simulink model "W05_1_vrx"  (R2024b)
settings: Solver=ode4  StartTime=0.0  StopTime=inf  FixedStep=Ts_ctrl  RelTol=1e-3
values from neighbouring files (symbols this model uses):
  animate = 0    [W05_compare.m]    (also in W05_crab_demo.m; W05_lookahead_demo.m; W05_setup.m = 1; W07_setup.m = 1)
  Delta = DELTAS(i)    [W05_lookahead_demo.m]    (also in W05_setup.m = 10; W07_setup.m = 10)
  F_max = 500    [W05_setup.m]    (also in W07_setup.m)
  guidance_mode = CASES{i,2}    [W05_compare.m]    (also in W05_setup.m = 2; W07_setup.m = 2)
  half_beam = 1.027135    [W05_setup.m]    (also in W07_setup.m)
  k_prop = 1000 * 0.004422 * 0.2^4    (= 0.0070752)    [W05_setup.m]    (also in W07_setup.m)
  Kd_psi = 200    [W05_setup.m]    (also in W07_setup.m)
  Ki_u = 100    [W05_setup.m]    (also in W07_setup.m)
  Kp_psi = 400    [W05_setup.m]    (also in W07_setup.m)
  Kp_u = 300    [W05_setup.m]    (also in W07_setup.m)
  n_max = sqrt(F_max / k_prop)    [W05_setup.m]    (also in W07_setup.m)
  origin_east = -532    [W05_setup.m]    (also in W07_setup.m)
  origin_north = 162    [W05_setup.m]    (also in W07_setup.m)
  R_LOS = 5    [W05_lookahead_demo.m]    (also in W05_setup.m; W07_setup.m)
  sw_mode = 1    [W05_lookahead_demo.m]    (also in W05_setup.m; W07_setup.m)
  tau_n = 0.30    (= 0.3)    [W05_setup.m]    (also in W07_setup.m)
  Ts_ctrl = 0.05    [W05_setup.m]    (also in W07_setup.m)
  u_ref = 1.5    [W05_setup.m]    (also in W07_setup.m)
  wp_east = [  20   20  100  100   20 ]    [W05_setup.m]    (also in W07_setup.m)
  wp_north = [ -20   60   60  -20  -20 ]    [W05_setup.m]    (also in W07_setup.m)
libraries: ros2lib x5, slpidlib x1
settings Model: Creator=admin  LastModifiedBy=admin

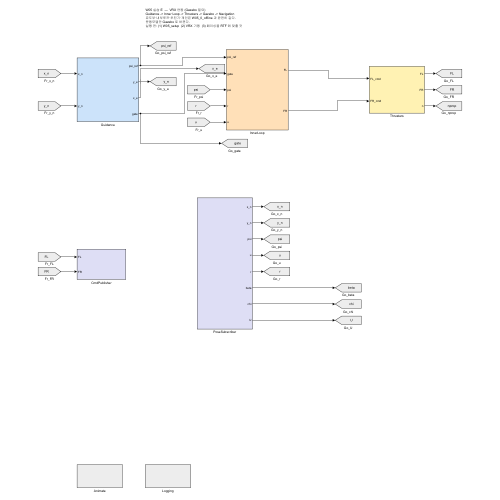
[thumbnail: Simulink's stored preview of the top-level diagram]
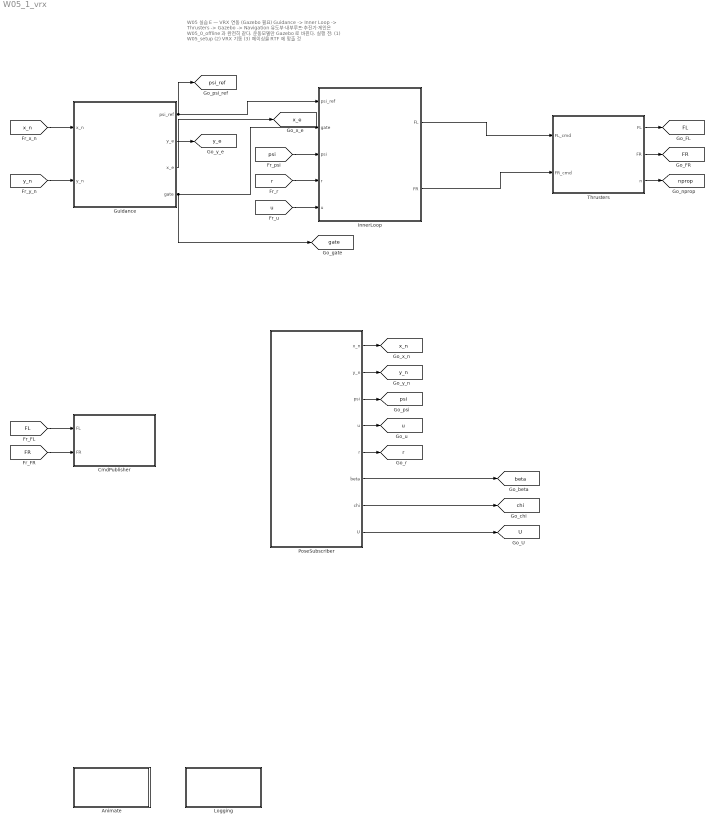
== system W05_1_vrx ==
  note: W05 실습 E  —  VRX 연동 (Gazebo 필요)
      | Guidance -> Inner Loop -> Thrusters -> Gazebo -> Navigation
      | 유도부·내부루프·추진기·게인은 W05_0_offline 과 완전히 같다.
      | 운동모델만 Gazebo 로 바뀐다.
      | 실행 전: (1) W05_setup  (2) VRX 기동  (3) 페이싱을 RTF 에 맞출 것
  Animate : Subsystem
  CmdPublisher : Subsystem
  Guidance : Subsystem
  InnerLoop : Subsystem
  Logging : Subsystem
  PoseSubscriber : Subsystem
  Thrusters : Subsystem
  tag scope: FL=global, FR=global, U=global, beta=global, chi=global, gate=global, nprop=global, psi=global, psi_ref=global, r=global, u=global, x_e=global, x_n=global, y_e=global, y_n=global
  wires:
  [FR] -> CmdPublisher/2(FR)
  [FL] -> CmdPublisher/1(FL)
  InnerLoop/2(FR) -> Thrusters/2(FR_cmd)
  InnerLoop/1(FL) -> Thrusters/1(FL_cmd)
  [u] -> InnerLoop/5(u)
  [r] -> InnerLoop/4(r)
  [psi] -> InnerLoop/3(psi)
  Guidance/4(gate) -> InnerLoop/2(gate), [gate]
  Guidance/1(psi_ref) -> InnerLoop/1(psi_ref), [psi_ref]
  [y_n] -> Guidance/2(y_n)
  [x_n] -> Guidance/1(x_n)
  Thrusters/1(FL) -> [FL]
  Thrusters/2(FR) -> [FR]
  PoseSubscriber/8(U) -> [U]
  PoseSubscriber/6(beta) -> [beta]
  PoseSubscriber/7(chi) -> [chi]
  Thrusters/3(n) -> [nprop]
  PoseSubscriber/3(psi) -> [psi]
  PoseSubscriber/5(r) -> [r]
  PoseSubscriber/4(u) -> [u]
  Guidance/3(x_e) -> [x_e]
  PoseSubscriber/1(x_n) -> [x_n]
  Guidance/2(y_e) -> [y_e]
  PoseSubscriber/2(y_n) -> [y_n]

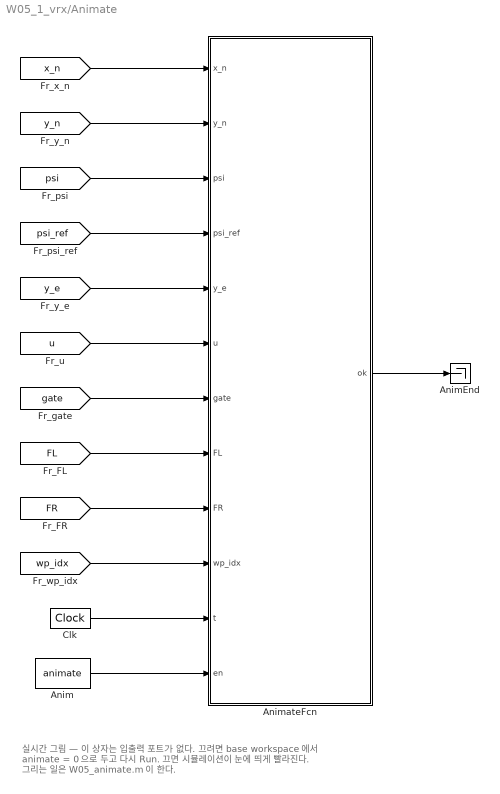
== system W05_1_vrx/Animate ==
  note: 실시간 그림 — 이 상자는 입출력 포트가 없다.
      | 끄려면 base workspace 에서  animate = 0  으로 두고 다시 Run.
      | 끄면 시뮬레이션이 눈에 띄게 빨라진다.
      | 그리는 일은 W05_animate.m 이 한다.
  Anim : Constant  Value=animate
  AnimEnd : Terminator
  AnimateFcn : MATLAB Function  TreatAsAtomicUnit=on
  Clk : DigitalClock  SampleTime=Ts_ctrl
  wires:
  [x_n] -> AnimateFcn/1(x_n)
  [y_n] -> AnimateFcn/2(y_n)
  [psi] -> AnimateFcn/3(psi)
  [psi_ref] -> AnimateFcn/4(psi_ref)
  [y_e] -> AnimateFcn/5(y_e)
  [u] -> AnimateFcn/6(u)
  [gate] -> AnimateFcn/7(gate)
  [FL] -> AnimateFcn/8(FL)
  [FR] -> AnimateFcn/9(FR)
  [wp_idx] -> AnimateFcn/10(wp_idx)
  Clk/1 -> AnimateFcn/11(t)
  Anim/1 -> AnimateFcn/12(en)
  AnimateFcn/1(ok) -> AnimEnd/1

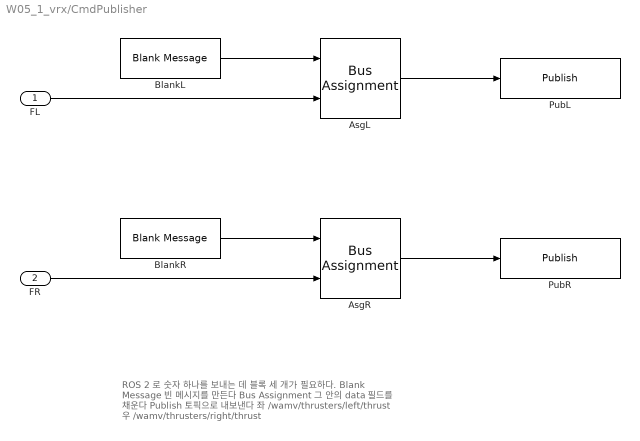
== system W05_1_vrx/CmdPublisher ==
  note: ROS 2 로 숫자 하나를 보내는 데 블록 세 개가 필요하다.
      |   Blank Message   빈 메시지를 만든다
      |   Bus Assignment  그 안의 data 필드를 채운다
      |   Publish         토픽으로 내보낸다
      |
      | 좌 /wamv/thrusters/left/thrust
      | 우 /wamv/thrusters/right/thrust
  FL : Inport
  FR : Inport  Port=2
  AsgL : BusAssignment  AssignedSignals=data
  AsgR : BusAssignment  AssignedSignals=data
  BlankL : ros2lib/Blank Message  messageClass=Message  entityType=std_msgs/Float64  messageType=std_msgs/Float64  SampleTime=Ts_ctrl
  BlankR : ros2lib/Blank Message  messageClass=Message  entityType=std_msgs/Float64  messageType=std_msgs/Float64  SampleTime=Ts_ctrl
  PubL : ros2lib/Publish  topicSource=Specify your own  topic=/wamv/thrusters/left/thrust  messageType=std_msgs/Float64  QOSHistory=Keep last  QOSDepth=1  QOSReliability=Reliable  QOSDurability=Volatile  QOSDeadline=Inf  QOSLifespan=Inf  QOSLiveliness=Automatic  QOSLeaseDuration=Inf  QOSAvoidROSNamespaceConventions=off
  PubR : ros2lib/Publish  topicSource=Specify your own  topic=/wamv/thrusters/right/thrust  messageType=std_msgs/Float64  QOSHistory=Keep last  QOSDepth=1  QOSReliability=Reliable  QOSDurability=Volatile  QOSDeadline=Inf  QOSLifespan=Inf  QOSLiveliness=Automatic  QOSLeaseDuration=Inf  QOSAvoidROSNamespaceConventions=off
  wires:
  BlankL/1 -> AsgL/1
  AsgL/1 -> PubL/1
  FL/1 -> AsgL/2
  BlankR/1 -> AsgR/1
  AsgR/1 -> PubR/1
  FR/1 -> AsgR/2

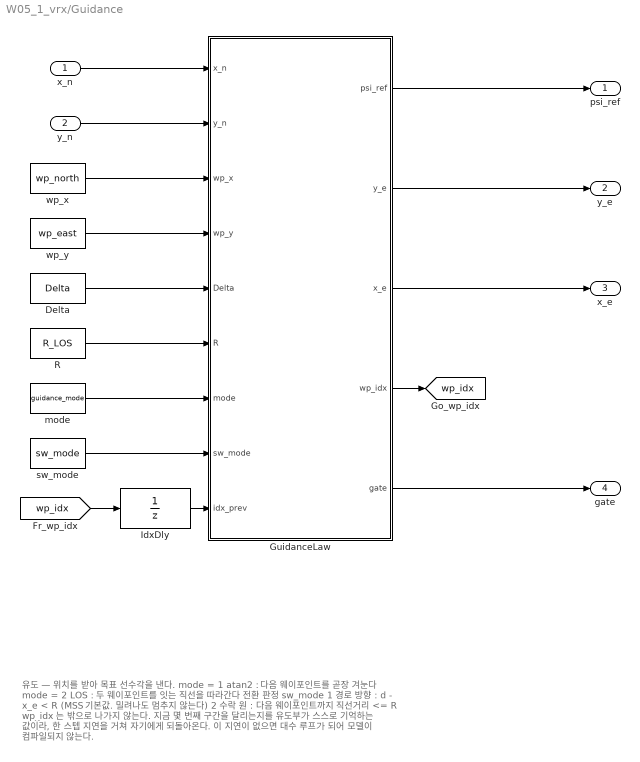
== system W05_1_vrx/Guidance ==
  note: 유도 — 위치를 받아 목표 선수각을 낸다.
      |   mode = 1  atan2 : 다음 웨이포인트를 곧장 겨눈다
      |   mode = 2  LOS   : 두 웨이포인트를 잇는 직선을 따라간다
      |
      | 전환 판정 sw_mode
      |   1  경로 방향 : d - x_e < R   (MSS 기본값. 밀려나도 멈추지 않는다)
      |   2  수락 원   : 다음 웨이포인트까지 직선거리 <= R
      |
      | wp_idx 는 밖으로 나가지 않는다. 지금 몇 번째 구간을 달리는지를
      | 유도부가 스스로 기억하는 값이라, 한 스텝 지연을 거쳐 자기에게 되돌아온다.
      | 이 지연이 없으면 대수 루프가 되어 모델이 컴파일되지 않는다.
  x_n : Inport
  y_n : Inport  Port=2
  Delta : Constant  Value=Delta
  GuidanceLaw : MATLAB Function  TreatAsAtomicUnit=on
  IdxDly : UnitDelay  Description=대수 루프 차단 + 사건 계수기 — 웨이포인트 번호는 정수이고, 유도부가 낸 값이 유도부로 되돌아온다. 미분방정식의 상태가 아니다.  InitialCondition=1  SampleTime=Ts_ctrl  HasFrameUpgradeWarning=on
  R : Constant  Value=R_LOS
  mode : Constant  Value=guidance_mode
  sw_mode : Constant  Value=sw_mode
  wp_x : Constant  Value=wp_north
  wp_y : Constant  Value=wp_east
  psi_ref : Outport
  y_e : Outport  Port=2
  x_e : Outport  Port=3
  gate : Outport  Port=4
  tag scope: wp_idx=global
  wires:
  x_n/1 -> GuidanceLaw/1(x_n)
  y_n/1 -> GuidanceLaw/2(y_n)
  wp_x/1 -> GuidanceLaw/3(wp_x)
  wp_y/1 -> GuidanceLaw/4(wp_y)
  Delta/1 -> GuidanceLaw/5(Delta)
  R/1 -> GuidanceLaw/6(R)
  mode/1 -> GuidanceLaw/7(mode)
  sw_mode/1 -> GuidanceLaw/8(sw_mode)
  [wp_idx] -> IdxDly/1
  IdxDly/1 -> GuidanceLaw/9(idx_prev)
  GuidanceLaw/1(psi_ref) -> psi_ref/1
  GuidanceLaw/2(y_e) -> y_e/1
  GuidanceLaw/3(x_e) -> x_e/1
  GuidanceLaw/5(gate) -> gate/1
  GuidanceLaw/4(wp_idx) -> [wp_idx]

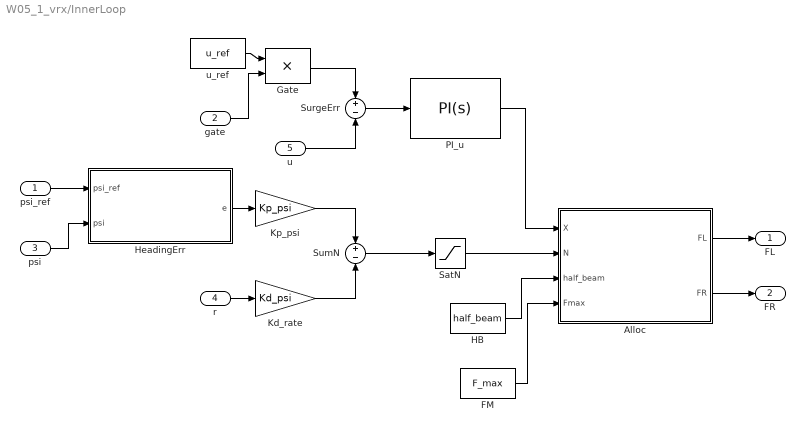
== system W05_1_vrx/InnerLoop ==
  psi_ref : Inport
  gate : Inport  Port=2
  psi : Inport  Port=3
  r : Inport  Port=4
  u : Inport  Port=5
  Alloc : MATLAB Function  TreatAsAtomicUnit=on
  FM : Constant  Value=F_max
  Gate : Product
  HB : Constant  Value=half_beam
  HeadingErr : MATLAB Function  TreatAsAtomicUnit=on
  Kd_rate : Gain  Gain=Kd_psi
  Kp_psi : Gain  Gain=Kp_psi
  PI_u : slpidlib/PID Controller  Controller=PI  Form=Parallel  TimeDomain=Continuous-time  UseExternalTs=off  SampleTime=-1  IntegratorMethod=Forward Euler  FilterMethod=Forward Euler  ControllerParametersSource=internal  P=Kp_u  I=Ki_u  UseKiTs=off  D=0  UseExternalDerivativeSource=off  N=100  UseFilter=on  TunerSelectOption=Transfer Function Based (PID Tuner App)  InitialConditionSource=internal  InitialConditionForIntegrator=0  InitialConditionForFilter=0  DifferentiatorICPrevScaledInput=0  ExternalReset=none  TrackingMode=off  Kt=1  LimitOutput=on  SatLimitsSource=internal  UpperSaturationLimit=2*F_max  LowerSaturationLimit=-2*F_max  LinearizeAsGain=on  AntiWindupMode=clamping  Kb=1  LimitIntegrator=off  UpperIntegratorSaturationLimit=inf  LowerIntegratorSaturationLimit=-inf  POutMin=[]  POutMax=[]  IOutMin=[]  IOutMax=[]  DOutMin=[]  DOutMax=[]  NOutMin=[]  NOutMax=[]  SumOutMin=[]  SumOutMax=[]  SaturationOutMin=[]  SaturationOutMax=[]  PParamMin=[]  PParamMax=[]  IParamMin=[]  IParamMax=[]  DParamMin=[]  DParamMax=[]  NParamMin=[]  NParamMax=[]  KbParamMin=[]  KbParamMax=[]  KtParamMin=[]  KtParamMax=[]  KbOutMin=[]  KbOutMax=[]  KtOutMin=[]  KtOutMax=[]  IntegratorOutMin=[]  IntegratorOutMax=[]  FilterOutMin=[]  FilterOutMax=[]  SumI1OutMin=[]  SumI1OutMax=[]  SumI2OutMin=[]  SumI2OutMax=[]  SumI3OutMin=[]  SumI3OutMax=[]  SumI4OutMin=[]  SumI4OutMax=[]  SumDOutMin=[]  SumDOutMax=[]  DifferentiatorOutMin=[]  DifferentiatorOutMax=[]  FilterDiffOutCoefMin=[]  FilterDiffOutCoefMax=[]  ReciprocalOutMin=[]  ReciprocalOutMax=[]  SumDenOutMin=[]  SumDenOutMax=[]  SumNumOutMin=[]  SumNumOutMax=[]  DivideOutMin=[]  DivideOutMax=[]  UdiffTsProdOutMin=[]  UdiffTsProdOutMax=[]  NTsProdOutMin=[]  NTsProdOutMax=[]  UintegralTsProdOutMin=[]  UintegralTsProdOutMax=[]  UngainTsProdOutMin=[]  UngainTsProdOutMax=[]  ClampingZeroOutDataTypeStr=Inherit: Inherit via back propagation  ClampingZeroOutMin=[]  ClampingZeroOutMax=[]  FilterDenConstantOutDataTypeStr=Inherit: Inherit via back propagation  FilterDenConstantOutMin=[]  FilterDenConstantOutMax=[]  PCopyOutDataTypeStr=Inherit: Inherit via back propagation  PCopyOutMin=[]  PCopyOutMax=[]  NCopyOutDataTypeStr=Inherit: Inherit via back propagation  NCopyOutMin=[]  NCopyOutMax=[]  IntegratorContinuousStateAttributes=''  IntegratorStateMustResolveToSignalObject=off  IntegratorRTWStateStorageClass=Auto  FilterContinuousStateAttributes=''  FilterStateMustResolveToSignalObject=off  FilterRTWStateStorageClass=Auto  ParallelPVariant=InternalParameters  IdealPVariant=Disabled  IVariant=InternalParameters  DVariant=Disabled  IntegratorVariant=Continuous  SatVariant=Enabled  AWVariant=ContClampingParallel  PCopyVariant=Disabled  TRVariant=Disabled  FdbkBlocksVariant=Forward  IdealPFdbkVariant=Disabled  SatFdbkVariant=Disabled  DerivativeFilterVariant=Disabled  NVariant=Disabled  NCopyVariant=Disabled_SignalSpec  FilterICVariant=Disabled  IntegratorICVariant=InternalICs  ExternalResetVariant=Disabled  TRSumVariant=Passthrough  SumFdbkVariant=Disabled  SumVariant=Sum_PI  TsampFilterVariant=InternalTs  TsampNgainVariant=Passthrough  TsampIntegralVariant=Disabled_SignalSpec  ExternalSaturationOutDataTypeStr=Inherit: Same as second input  DerivativeSourceVariant=Disabled  PreIntVariant=InternalPreInt
  SatN : Saturate  UpperLimit=2*F_max*half_beam  LowerLimit=-2*F_max*half_beam
  SumN : Sum  Inputs=+-
  SurgeErr : Sum  Inputs=+-
  u_ref : Constant  Value=u_ref
  FL : Outport
  FR : Outport  Port=2
  wires:
  psi_ref/1 -> HeadingErr/1(psi_ref)
  HeadingErr/1(e) -> Kp_psi/1
  u/1 -> SurgeErr/2
  Gate/1 -> SurgeErr/1
  psi/1 -> HeadingErr/2(psi)
  u_ref/1 -> Gate/1
  HB/1 -> Alloc/3(half_beam)
  gate/1 -> Gate/2
  r/1 -> Kd_rate/1
  Kp_psi/1 -> SumN/1
  Kd_rate/1 -> SumN/2
  SurgeErr/1 -> PI_u/1
  SumN/1 -> SatN/1
  PI_u/1 -> Alloc/1(X)
  SatN/1 -> Alloc/2(N)
  FM/1 -> Alloc/4(Fmax)
  Alloc/1(FL) -> FL/1
  Alloc/2(FR) -> FR/1

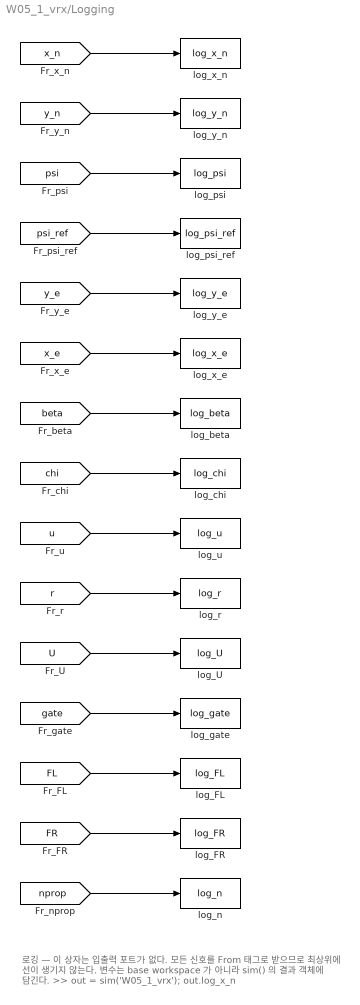
== system W05_1_vrx/Logging ==
  note: 로깅 — 이 상자는 입출력 포트가 없다.
      | 모든 신호를 From 태그로 받으므로 최상위에 선이 생기지 않는다.
      | 변수는 base workspace 가 아니라 sim() 의 결과 객체에 담긴다.
      |   >> out = sim('W05_1_vrx');  out.log_x_n
  log_FL : ToWorkspace  VariableName=log_FL  SaveFormat=Timeseries  SampleTime=Ts_ctrl
  log_FR : ToWorkspace  VariableName=log_FR  SaveFormat=Timeseries  SampleTime=Ts_ctrl
  log_U : ToWorkspace  VariableName=log_U  SaveFormat=Timeseries  SampleTime=Ts_ctrl
  log_beta : ToWorkspace  VariableName=log_beta  SaveFormat=Timeseries  SampleTime=Ts_ctrl
  log_chi : ToWorkspace  VariableName=log_chi  SaveFormat=Timeseries  SampleTime=Ts_ctrl
  log_gate : ToWorkspace  VariableName=log_gate  SaveFormat=Timeseries  SampleTime=Ts_ctrl
  log_n : ToWorkspace  VariableName=log_n  SaveFormat=Timeseries  SampleTime=Ts_ctrl
  log_psi : ToWorkspace  VariableName=log_psi  SaveFormat=Timeseries  SampleTime=Ts_ctrl
  log_psi_ref : ToWorkspace  VariableName=log_psi_ref  SaveFormat=Timeseries  SampleTime=Ts_ctrl
  log_r : ToWorkspace  VariableName=log_r  SaveFormat=Timeseries  SampleTime=Ts_ctrl
  log_u : ToWorkspace  VariableName=log_u  SaveFormat=Timeseries  SampleTime=Ts_ctrl
  log_x_e : ToWorkspace  VariableName=log_x_e  SaveFormat=Timeseries  SampleTime=Ts_ctrl
  log_x_n : ToWorkspace  VariableName=log_x_n  SaveFormat=Timeseries  SampleTime=Ts_ctrl
  log_y_e : ToWorkspace  VariableName=log_y_e  SaveFormat=Timeseries  SampleTime=Ts_ctrl
  log_y_n : ToWorkspace  VariableName=log_y_n  SaveFormat=Timeseries  SampleTime=Ts_ctrl
  wires:
  [x_n] -> log_x_n/1
  [y_n] -> log_y_n/1
  [psi] -> log_psi/1
  [psi_ref] -> log_psi_ref/1
  [y_e] -> log_y_e/1
  [x_e] -> log_x_e/1
  [beta] -> log_beta/1
  [chi] -> log_chi/1
  [u] -> log_u/1
  [r] -> log_r/1
  [U] -> log_U/1
  [gate] -> log_gate/1
  [FL] -> log_FL/1
  [FR] -> log_FR/1
  [nprop] -> log_n/1

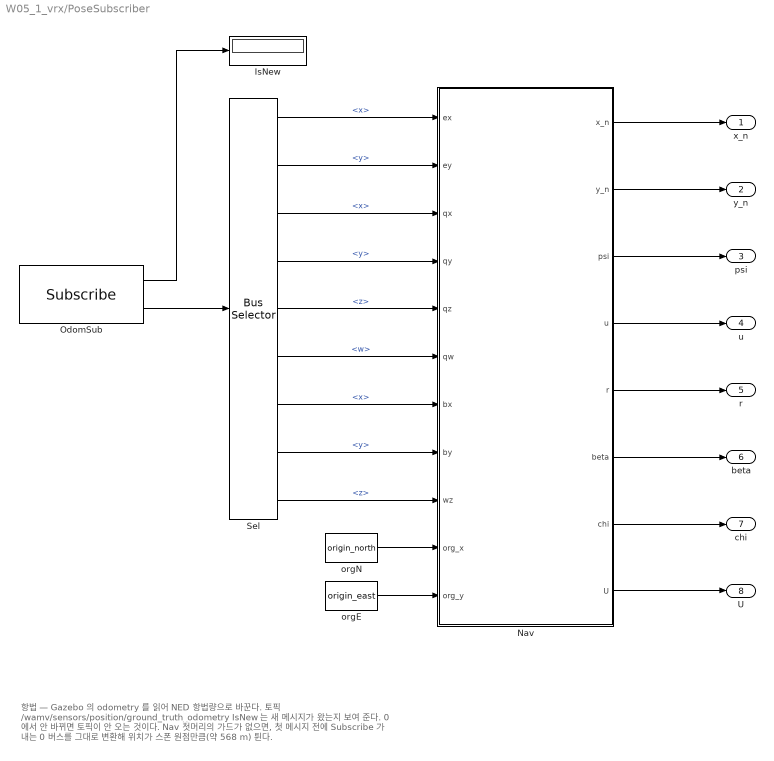
== system W05_1_vrx/PoseSubscriber ==
  note: 항법 — Gazebo 의 odometry 를 읽어 NED 항법량으로 바꾼다.
      |   토픽 /wamv/sensors/position/ground_truth_odometry
      |
      | IsNew 는 새 메시지가 왔는지 보여 준다. 0 에서 안 바뀌면 토픽이 안 오는 것이다.
      | Nav 첫머리의 가드가 없으면, 첫 메시지 전에 Subscribe 가 내는 0 버스를
      | 그대로 변환해 위치가 스폰 원점만큼(약 568 m) 튄다.
  IsNew : Display
  Nav : MATLAB Function  TreatAsAtomicUnit=on
  OdomSub : ros2lib/Subscribe  topicSource=Specify your own  topic=/wamv/sensors/position/ground_truth_odometry  messageType=nav_msgs/Odometry  sampleTime=Ts_ctrl  QOSHistory=Keep last  QOSDepth=1  QOSReliability=Reliable  QOSDurability=Volatile  QOSDeadline=Inf  QOSLifespan=Inf  QOSLiveliness=Automatic  QOSLeaseDuration=Inf  QOSAvoidROSNamespaceConventions=off
  Sel : BusSelector  OutputSignals=pose.pose.position.x,pose.pose.position.y,pose.pose.orientation.x,pose.pose.orientation.y,pose.pose.orientation.z,pose.pose.orientation.w,twist.twist.linear.x,twist.twist.linear.y,twist.twist.angular.z
  orgE : Constant  Value=origin_east
  orgN : Constant  Value=origin_north
  x_n : Outport
  y_n : Outport  Port=2
  psi : Outport  Port=3
  u : Outport  Port=4
  r : Outport  Port=5
  beta : Outport  Port=6
  chi : Outport  Port=7
  U : Outport  Port=8
  wires:
  OdomSub/1 -> IsNew/1
  OdomSub/2 -> Sel/1
  Sel/1 -> Nav/1(ex)  "<x>"
  Sel/2 -> Nav/2(ey)  "<y>"
  Sel/3 -> Nav/3(qx)  "<x>"
  Sel/4 -> Nav/4(qy)  "<y>"
  Sel/5 -> Nav/5(qz)  "<z>"
  Sel/6 -> Nav/6(qw)  "<w>"
  Sel/7 -> Nav/7(bx)  "<x>"
  Sel/8 -> Nav/8(by)  "<y>"
  Sel/9 -> Nav/9(wz)  "<z>"
  orgN/1 -> Nav/10(org_x)
  orgE/1 -> Nav/11(org_y)
  Nav/1(x_n) -> x_n/1
  Nav/2(y_n) -> y_n/1
  Nav/3(psi) -> psi/1
  Nav/4(u) -> u/1
  Nav/5(r) -> r/1
  Nav/6(beta) -> beta/1
  Nav/7(chi) -> chi/1
  Nav/8(U) -> U/1

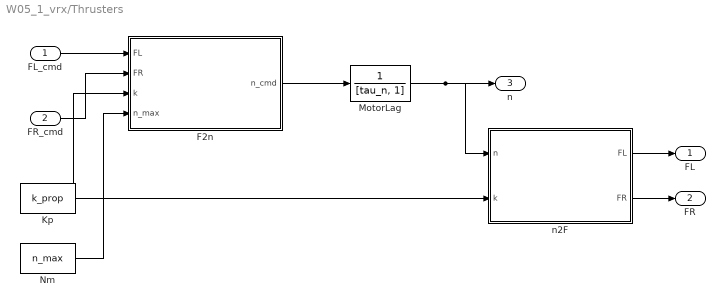
== system W05_1_vrx/Thrusters ==
  FL_cmd : Inport
  FR_cmd : Inport  Port=2
  F2n : MATLAB Function  TreatAsAtomicUnit=on
  Kp : Constant  Value=k_prop
  MotorLag : TransferFcn  Numerator=1  Denominator=[tau_n, 1]
  Nm : Constant  Value=n_max
  n2F : MATLAB Function  TreatAsAtomicUnit=on
  FL : Outport
  FR : Outport  Port=2
  n : Outport  Port=3
  wires:
  FL_cmd/1 -> F2n/1(FL)
  Nm/1 -> F2n/4(n_max)
  FR_cmd/1 -> F2n/2(FR)
  n2F/1(FL) -> FL/1
  MotorLag/1 -> n2F/1(n), n/1
  Kp/1 -> n2F/2(k), F2n/3(k)
  F2n/1(n_cmd) -> MotorLag/1
  n2F/2(FR) -> FR/1

== matlab function W05_1_vrx/Animate/AnimateFcn ==
  data: x_n input; y_n input; psi input; psi_ref input; y_e input; u input; ok output; gate input; FL input; FR input; wp_idx input; t input; en input
function ok = AnimateFcn(x_n, y_n, psi, psi_ref, y_e, u, gate, FL, FR, wp_idx, t, en)
%#codegen
% Live plot while the model runs. A MATLAB Function block cannot
% plot, so the drawing function is declared extrinsic: Simulink
% calls plain MATLAB instead of generating code for it.
coder.extrinsic('W05_animate');
ok = 1;
if en > 0.5
    W05_animate(x_n, y_n, psi, psi_ref, y_e, u, gate, FL, FR, wp_idx, t);
end

== matlab function W05_1_vrx/InnerLoop/HeadingErr ==
  data: psi_ref input; e output; psi input
function e = HeadingErr(psi_ref, psi)
%#codegen
% Shortest signed angle (ssa). Without it a command of 179 deg
% against a heading of -179 deg reads as a 358 deg error and
% the boat turns the long way round.
d = psi_ref - psi;
e = atan2(sin(d), cos(d));

== matlab function W05_1_vrx/Guidance/GuidanceLaw ==
  data: x_n input; psi_ref output; y_n input; wp_x input; wp_y input; Delta input; R input; mode input; sw_mode input; idx_prev input; y_e output; x_e output; wp_idx output; gate output
function [psi_ref, y_e, x_e, wp_idx, gate] = GuidanceLaw(x_n, y_n, wp_x, wp_y, Delta, R, mode, sw_mode, idx_prev)
%#codegen
% Waypoint guidance. Two laws in one block. Both return a HEADING command,
% following the MSS demo demoOtterUSVHeadingControl.slx and GNC/LOSchi.m.
%   mode 1 = atan2 : aim straight at the next waypoint (point chasing)
%   mode 2 = LOS   : follow the straight line between two waypoints
% Switching criterion (sw_mode):
%   1 = along-track : d - x_e < R      (MSS / Fossen default, cannot hang)
%   2 = circle      : distance to the next waypoint <= R

n = numel(wp_x);
k = min(max(idx_prev, 1), n-1);        % index of the active leg

xk  = wp_x(k);    yk  = wp_y(k);       % leg start
xk1 = wp_x(k+1);  yk1 = wp_y(k+1);     % leg end = next waypoint

% path-tangential angle of the active leg, measured from North
pi_p = atan2(yk1 - yk, xk1 - xk);

% Both errors come out of ONE rotation of (p - p_k) into the path frame.
% x_e = how far ALONG the leg,  y_e = how far TO THE SIDE of it.
% Computed the same way for BOTH guidance laws so that the two can be
% compared with the same yardstick.
x_e =  (x_n - xk)*cos(pi_p) + (y_n - yk)*sin(pi_p);
y_e = -(x_n - xk)*sin(pi_p) + (y_n - yk)*cos(pi_p);

if mode == 1
    psi_ref = atan2(yk1 - y_n, xk1 - x_n);
else
    psi_ref = pi_p - atan(y_e / Delta);
end

% --- waypoint switching ---------------------------------------------
% d is the leg length, so d - x_e is the along-track distance REMAINING.
% The circle test is always the stricter of the two, because
%     distance = sqrt((d - x_e)^2 + y_e^2) >= d - x_e
% A boat blown wide of a waypoint never enters that circle, and a mission
% that waits for it waits for ever. The along-track test cannot hang.
d = sqrt((xk1 - xk)^2 + (yk1 - yk)^2);
if sw_mode == 1
    reached = (d - x_e) < R;
else
    reached = sqrt((xk1 - x_n)^2 + (yk1 - y_n)^2) <= R;
end

% wp_idx = n means "mission finished" and it LATCHES: once the last leg is
% done, the boat stays stopped even if the current pushes it back behind the
% finish line (then reached would turn false again).
if idx_prev >= n
    wp_idx = n;                         % already finished - stay finished
elseif reached && (k < n-1)
    wp_idx = k + 1;
elseif reached && (k == n-1)
    wp_idx = n;                         % last leg done
else
    wp_idx = k;
end

% gate = 0 brings the boat to a stop. Without it the boat would follow the
% last leg forever.
gate = double(wp_idx < n);

== matlab function W05_1_vrx/InnerLoop/Alloc ==
  data: X input; FL output; N input; half_beam input; Fmax input; FR output
function [FL, FR] = Alloc(X, N, half_beam, Fmax)
%#codegen
% Differential thrust allocation for two aft thrusters.
%   X = FL + FR              surge force [N]
%   N = (FL - FR)*half_beam  yaw moment  [N*m]
FL = X/2 + N/(2*half_beam);
FR = X/2 - N/(2*half_beam);
if FL >  Fmax, FL =  Fmax; end
if FL < -Fmax, FL = -Fmax; end
if FR >  Fmax, FR =  Fmax; end
if FR < -Fmax, FR = -Fmax; end

== matlab function W05_1_vrx/Thrusters/F2n ==
  data: FL input; n_cmd output; FR input; k input; n_max input
function n_cmd = F2n(FL, FR, k, n_max)
%#codegen
% Inverse propeller law: turn a demanded thrust into a shaft speed.
%   F = k*n*|n|   ->   n = sign(F)*sqrt(|F|/k)
% Saturation happens on SPEED, not on force. That is what a real
% motor limits.
F = [FL; FR];
n_cmd = zeros(2,1);
for i = 1:2
    ni = sign(F(i)) * sqrt(abs(F(i))/k);
    if ni >  n_max, ni =  n_max; end
    if ni < -n_max, ni = -n_max; end
    n_cmd(i) = ni;
end

== matlab function W05_1_vrx/Thrusters/n2F ==
  data: n input; FL output; k input; FR output
function [FL, FR] = n2F(n, k)
%#codegen
% Forward propeller law. Note the |n| : thrust is quadratic in
% shaft speed, so a rate limit on n is NOT a rate limit on F.
FL = k * n(1) * abs(n(1));
FR = k * n(2) * abs(n(2));

== matlab function W05_1_vrx/PoseSubscriber/Nav ==
  data: ex input; x_n output; ey input; qx input; qy input; qz input; qw input; bx input; by input; wz input; org_x input; org_y input; y_n output; psi output; u output; r output; beta output; chi output; U output
function [x_n, y_n, psi, u, r, beta, chi, U] = Nav(ex, ey, qx, qy, qz, qw, bx, by, wz, org_x, org_y)
%#codegen
% Gazebo/ROS uses ENU with a body frame of x-forward, y-LEFT, z-UP.
% Marine control uses NED with a body frame of x-forward, y-STARBOARD.
% Position :  N = y_ENU,  E = x_ENU
% Heading  :  psi_NED = pi/2 - yaw_ENU
% Body vel :  u = bx,  v = -by,  r = -wz    (y and z flip sign)

% 첫 메시지가 도착하기 전에는 Subscribe 가 0 으로 채운 버스를 낸다.
% 그대로 쓰면 위치가 스폰 원점만큼(약 568 m) 튀어 로그 첫 점이 망가진다.
if ex == 0 && ey == 0
    x_n = 0; y_n = 0; psi = 0; u = 0; r = 0; beta = 0; chi = 0; U = 0;
    return
end
x_n = ey - org_x;    % north, relative to the spawn point
y_n = ex - org_y;    % east

yaw_enu = atan2(2*(qw*qz + qx*qy), 1 - 2*(qy*qy + qz*qz));
p   = pi/2 - yaw_enu;
psi = atan2(sin(p), cos(p));

u = bx;
v = -by;
r = -wz;

U    = sqrt(u*u + v*v);
beta = atan2(v, u);          % crab angle
c    = psi + beta;
chi  = atan2(sin(c), cos(c));
